simulink model "my_cpm"  (R2014b)
settings: Solver=ode45  StartTime=0.0  StopTime=.5  RelTol=1e-3
libraries: commchan3 x4, simulink x4, commdigbbndcpm2 x2, dsparch4 x2, commrflib2 x2, commsink2 x1, siglabs_lib x1, commrandsrc2 x1, dspnetwork x1
settings Model: NumberOfSteps=500  SnapshotBufferSize=1000  Creator=Ben  LastModifiedBy=Ben

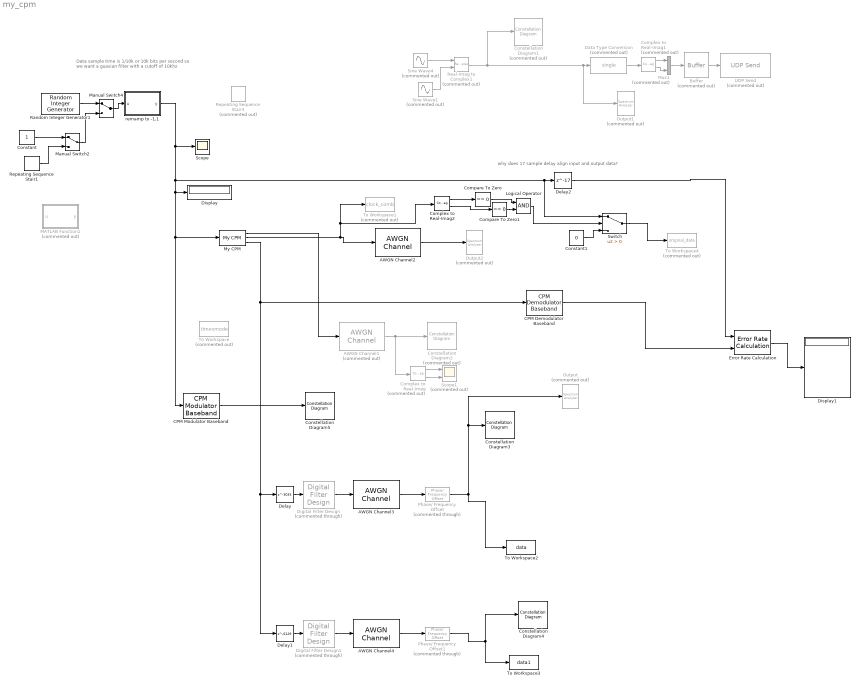
== system my_cpm ==
  note: why does 17 sample delay align input and output data?
  note: Data sample time is 1/10k or 10k bits per second
      | so we want a guasian filter with a cutoff of 10khz
  AWGN Channel1 : commchan3/AWGN Channel  Commented=on  InputProcessing=Columns as channels (frame based)  seed=67  noiseMode="Signal to noise ratio  (Eb/No)"  EbNodB=80  EsNodB=10  SNRdB=10  bitsPerSym=1  Ps=1  Tsym=1  variance=1
  AWGN Channel2 : commchan3/AWGN Channel  InputProcessing=Columns as channels (frame based)  seed=67  noiseMode="Signal to noise ratio  (SNR)"  EbNodB=80  EsNodB=10  SNRdB=40  bitsPerSym=1  Ps=1  Tsym=1  variance=1
  AWGN Channel3 : commchan3/AWGN Channel  InputProcessing=Columns as channels (frame based)  seed=67  noiseMode="Signal to noise ratio  (SNR)"  EbNodB=80  EsNodB=10  SNRdB=2  bitsPerSym=1  Ps=1  Tsym=1  variance=1
  AWGN Channel4 : commchan3/AWGN Channel  InputProcessing=Columns as channels (frame based)  seed=43  noiseMode="Signal to noise ratio  (SNR)"  EbNodB=80  EsNodB=10  SNRdB=2  bitsPerSym=1  Ps=1  Tsym=1  variance=1
  Buffer : Buffer  Commented=on  N=180  TreatMby1Signals=One channel
  CPM Demodulator Baseband : commdigbbndcpm2/CPM Demodulator Baseband  Mnum=2  outputType=Integer  mappingType=Binary  modIdx=2  pulseShape=Rectangular  BT=0.3  mainLobePulseLength=1  rollOff=0.2  pulseLength=1  preHistory=1  phaseOffset=0  samplesPerSymbol=10  RateOptions=Allow multirate processing  traceBack=16  outDType=double
  CPM Modulator Baseband : commdigbbndcpm2/CPM Modulator Baseband  Mnum=2  inputType=Integer  mappingType=Binary  modIdx=2  pulseShape=Rectangular  BT=0  mainLobePulseLength=1  rollOff=0.2  pulseLength=1  preHistory=1  phaseOffset=0  samplesPerSymbol=10  RateOptions=Allow multirate processing  outDataType=double
  Compare To Zero : simulink/Logic and Bit Operations/Compare To Zero  relop===  OutDataTypeStr=uint8
  Compare To Zero1 : simulink/Logic and Bit Operations/Compare To Zero  relop===  OutDataTypeStr=uint8
  Complex to Real-Imag : ComplexToRealImag  Commented=on
  Complex to Real-Imag1 : ComplexToRealImag  Commented=on
  Complex to Real-Imag2 : ComplexToRealImag
  Constant : Constant  SampleTime=1/(10000)
  Constant1 : Constant  Value=0
  Constellation Diagram1 : ConstellationDiagram  Commented=on
  Constellation Diagram2 : ConstellationDiagram  Commented=on
  Constellation Diagram3 : ConstellationDiagram
  Constellation Diagram4 : ConstellationDiagram
  Constellation Diagram5 : ConstellationDiagram
  Data Type Conversion : DataTypeConversion  Commented=on  OutDataTypeStr=single
  Delay : Delay  DelayLength=3033  InitialCondition=0
  Delay1 : Delay  DelayLength=6129  InitialCondition=0
  Delay2 : Delay  DelayLength=17  InitialCondition=0
  Digital Filter Design : dsparch4/Digital Filter Design  Commented=through  mwdsp_browser_bugfix_var=off
  Digital Filter Design1 : dsparch4/Digital Filter Design  Commented=through  mwdsp_browser_bugfix_var=off
  Display : Display
  Display1 : Display
  Error Rate Calculation : commsink2/Error Rate Calculation  N=0  st_delay=0  cp_mode=Entire frame  subframe=[]  PMode=Port  WsName=ErrorVec  RsMode2=off  stop=off  numErr=100  maxBits=1e6
  Logical Operator : Logic  AllPortsSameDT=off  OutDataTypeStr=boolean
  MATLAB Function1 : MATLAB Function  Commented=on  TreatAsAtomicUnit=on
  Manual Switch2 : ManualSwitch
  Manual Switch4 : ManualSwitch
  Mux1 : Mux  Commented=on  Inputs=2
  My CPM : siglabs_lib/My CPM  SampsPerSym=10
  Output : SpectrumAnalyzer  Commented=on
  Output1 : SpectrumAnalyzer  Commented=on
  Output2 : SpectrumAnalyzer  Commented=on
  Phase/ Frequency Offset : commrflib2/Phase// Frequency Offset  Commented=through  phaseOffset=42  freqPort=off  freqOffset=0
  Phase/ Frequency Offset1 : commrflib2/Phase// Frequency Offset  Commented=through  phaseOffset=42  freqPort=off  freqOffset=0
  Random Integer Generator1 : commrandsrc2/Random Integer Generator  mul=2  seed=42  Ts=1/(10000)  frameBased=off  sampPerFrame=1024  orient=off  outDataType=double
  Real-Imag to Complex1 : RealImagToComplex  Commented=on
  Repeating Sequence Stair1 : simulink/Sources/Repeating Sequence Stair  OutValues=[0 1].'  tsamp=1/(10000)  OutMin=[]  OutMax=[]  OutDataTypeStr=double  OutputDataTypeScalingMode=double  OutDataType=fixdt(0,8)  ConRadixGroup=Best Precision: Vector-wise  OutScaling=2^-12
  Repeating Sequence Stair3 : simulink/Sources/Repeating Sequence Stair  Commented=on  OutValues=[4 5 5 4].'  tsamp=0.00000002  OutMin=[]  OutMax=[]  OutDataTypeStr=double  OutputDataTypeScalingMode=double  OutDataType=fixdt(0,8)  ConRadixGroup=Best Precision: Vector-wise  OutScaling=2^-12
  Scope : Scope
      settings: YMin=-0  YMax=1
  Scope1 : Scope  Commented=on  NumInputPorts=2
      settings: TimeRange=0.1  YMin=-5~-5  YMax=5~5
  Sine Wave1 : Sin  Commented=on  Frequency=12.801*2*pi*1000  Phase=-pi/2  SampleTime=1/128000
  Sine Wave4 : Sin  Commented=on  Frequency=12.801*2*pi*1000  SampleTime=1/128000
  Switch : Switch  Criteria=u2 > Threshold
  To Workspace : ToWorkspace  Commented=on  VariableName=timevmode  SampleTime=-1
      settings: Save2DSignal=2-D array (concatenate along first dimension)
  To Workspace1 : ToWorkspace  Commented=on  VariableName=clock_comb  SampleTime=-1
      settings: Save2DSignal=2-D array (concatenate along first dimension)
  To Workspace2 : ToWorkspace  VariableName=data  SampleTime=-1
      settings: Save2DSignal=2-D array (concatenate along first dimension)
  To Workspace3 : ToWorkspace  VariableName=data1  SampleTime=-1
      settings: Save2DSignal=2-D array (concatenate along first dimension)
  To Workspace4 : ToWorkspace  Commented=on  VariableName=original_data  SampleTime=-1
      settings: Save2DSignal=2-D array (concatenate along first dimension)
  UDP Send : dspnetwork/UDP Send  Commented=on  remoteURL='192.168.1.13'  remotePort=25000  localURL='0.0.0.0'  localPortSource=Automatically determine  localPort=-1  sampletime=-1  separateLengthPort=0
  remamp to -1,1 : MATLAB Function  TreatAsAtomicUnit=on
  wires:
  AWGN Channel1/1 -> Complex to Real-Imag/1, Constellation Diagram2/1
  Complex to Real-Imag/1 -> Scope1/1
  Complex to Real-Imag/2 -> Scope1/2
  My CPM/1 -> AWGN Channel1/1
  Digital Filter Design/1 -> AWGN Channel3/1
  Manual Switch4/1 -> remamp to -1,1/1(u)
  Random Integer Generator1/1 -> Manual Switch4/1
  remamp to -1,1/1(y) -> Switch/1, Delay2/1, CPM Modulator Baseband/1, My CPM/1, Display/1, Scope/1
  Data Type Conversion/1 -> Complex to Real-Imag1/1
  Complex to Real-Imag1/1 -> Mux1/1
  Complex to Real-Imag1/2 -> Mux1/2
  Mux1/1 -> Buffer/1
  Buffer/1 -> UDP Send/1
  Repeating Sequence Stair1/1 -> Manual Switch2/2
  Constant/1 -> Manual Switch2/1
  Manual Switch2/1 -> Manual Switch4/2
  Sine Wave4/1 -> Real-Imag to Complex1/1
  Sine Wave1/1 -> Real-Imag to Complex1/2
  CPM Modulator Baseband/1 -> Constellation Diagram5/1
  Real-Imag to Complex1/1 -> Output1/1, Data Type Conversion/1, Constellation Diagram1/1
  My CPM/2 -> Complex to Real-Imag2/1, To Workspace1/1, AWGN Channel2/1
  My CPM/3 -> Delay1/1, Delay/1, CPM Demodulator Baseband/1
  AWGN Channel2/1 -> Output2/1
  AWGN Channel3/1 -> Phase/ Frequency Offset/1
  Phase/ Frequency Offset/1 -> Output/1, Constellation Diagram3/1, To Workspace2/1
  Delay/1 -> Digital Filter Design/1
  Error Rate Calculation/1 -> Display1/1
  Digital Filter Design1/1 -> AWGN Channel4/1
  AWGN Channel4/1 -> Phase/ Frequency Offset1/1
  Phase/ Frequency Offset1/1 -> Constellation Diagram4/1, To Workspace3/1
  Delay1/1 -> Digital Filter Design1/1
  CPM Demodulator Baseband/1 -> Error Rate Calculation/2
  Delay2/1 -> Error Rate Calculation/1
  Complex to Real-Imag2/1 -> Compare To Zero/1
  Complex to Real-Imag2/2 -> Compare To Zero1/1
  Compare To Zero1/1 -> Logical Operator/2
  Compare To Zero/1 -> Logical Operator/1
  Logical Operator/1 -> Switch/2
  Switch/1 -> To Workspace4/1
  Constant1/1 -> Switch/3

== matlab function my_cpm/remamp to -1,1 ==
  data: u input; y output
function y = fcn(u)
%#codegen

y = (u*2)-1;

== matlab function my_cpm/MATLAB Function1 ==
  data: u input; y output
function y = fcn(u)
%#codegen

y = u;
